simulink subsystem "Tank_system"  (R2020b)
settings: Solver=VariableStepAuto  StartTime=0.0  StopTime=10.0  RelTol=1e-3
libraries: simulink x5
settings Model: Creator=avina  LastModifiedBy=avina

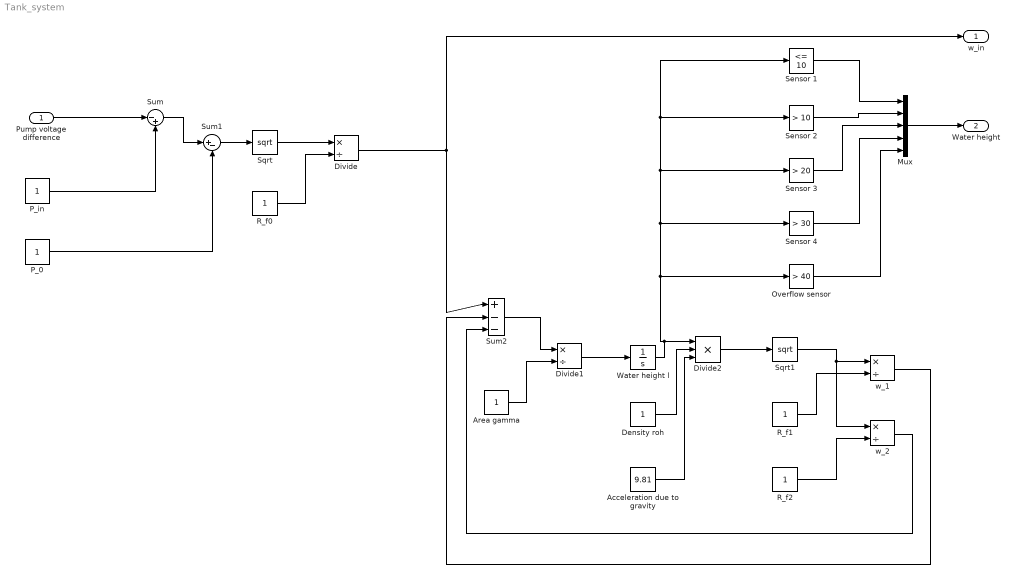
== system Tank_system ==
  Pump voltage difference : Inport
  Acceleration due to gravity : Constant  Value=9.81
  Area gamma : Constant
  Density roh : Constant
  Divide : Product  Inputs=*/
  Divide1 : Product  Inputs=*/
  Divide2 : Product  Inputs=***
  Mux : Mux  Inputs=5
  Overflow sensor : simulink/Logic and Bit Operations/Compare To Constant  relop=>  const=40  OutDataTypeStr=boolean
  P_0 : Constant
  P_in : Constant
  R_f0 : Constant
  R_f1 : Constant
  R_f2 : Constant
  Sensor 1 : simulink/Logic and Bit Operations/Compare To Constant  relop=<=  const=10  OutDataTypeStr=boolean
  Sensor 2 : simulink/Logic and Bit Operations/Compare To Constant  relop=>  const=10  OutDataTypeStr=boolean
  Sensor 3 : simulink/Logic and Bit Operations/Compare To Constant  relop=>  const=20  OutDataTypeStr=boolean
  Sensor 4 : simulink/Logic and Bit Operations/Compare To Constant  relop=>  const=30  OutDataTypeStr=boolean
  Sqrt : Sqrt  SaturateOnIntegerOverflow=on
  Sqrt1 : Sqrt  SaturateOnIntegerOverflow=on
  Sum : Sum  Inputs=|-+
  Sum1 : Sum  Inputs=|+-
  Sum2 : Sum  Inputs=|+--
  Water height l : Integrator
  w_1 : Product  Inputs=*/
  w_2 : Product  Inputs=*/
  w_in : Outport
  Water height : Outport  Port=2
  wires:
  Pump voltage difference/1 -> Sum/1
  P_in/1 -> Sum/2
  Sum/1 -> Sum1/1
  P_0/1 -> Sum1/2
  Sum1/1 -> Sqrt/1
  Sqrt/1 -> Divide/1
  R_f0/1 -> Divide/2
  Divide/1 -> w_in/1, Sum2/1
  Sum2/1 -> Divide1/1
  Area gamma/1 -> Divide1/2
  Divide1/1 -> Water height l/1
  Water height l/1 -> Divide2/1, Overflow sensor/1, Sensor 4/1, Sensor 1/1, Sensor 2/1, Sensor 3/1
  Density roh/1 -> Divide2/2
  Acceleration due to gravity/1 -> Divide2/3
  Divide2/1 -> Sqrt1/1
  Sqrt1/1 -> w_1/1, w_2/1
  R_f1/1 -> w_1/2
  R_f2/1 -> w_2/2
  w_2/1 -> Sum2/3
  w_1/1 -> Sum2/2
  Sensor 1/1 -> Mux/1
  Sensor 2/1 -> Mux/2
  Sensor 3/1 -> Mux/3
  Sensor 4/1 -> Mux/4
  Overflow sensor/1 -> Mux/5
  Mux/1 -> Water height/1
